simulink model "simu_test_2x1spokodziala1"  (Simulink 7.7)
settings: Solver=ode45  StartTime=0.0  StopTime=20.0  RelTol=1e-3
libraries: fuzblock x1, simulink x1
settings Model: Creator=Marcin  LastModifiedBy=Marcin

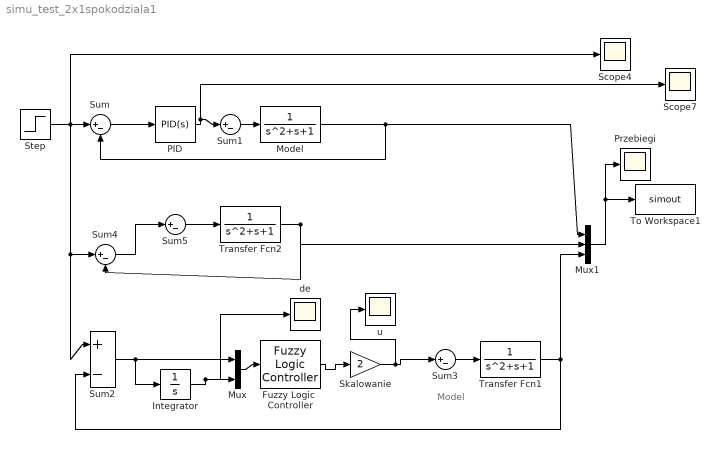
== system simu_test_2x1spokodziala1 ==
  note: Model
  Fuzzy Logic  Controller : fuzblock/Fuzzy Logic  Controller  SystemSampleTime=-1  fis=fls
  Integrator : Integrator
  Model : TransferFcn  Denominator=[1 1 1]
  Mux : Mux  Inputs=2
  Mux1 : Mux  Inputs=3
  PID : simulink/Continuous/PID Controller  SystemSampleTime=-1  Controller=PID  TimeDomain=Continuous-time  SampleTime=1  IntegratorMethod=Forward Euler  FilterMethod=Forward Euler  Form=Parallel  P=1  I=0.3  D=1  N=100  InitialConditionSource=internal  InitialConditionForIntegrator=0  InitialConditionForFilter=0  ExternalReset=none  LimitOutput=off  UpperSaturationLimit=inf  LowerSaturationLimit=-inf  LinearizeAsGain=off  AntiWindupMode=none  Kb=1  TrackingMode=off  Kt=1  PParamMin=[]  PParamMax=[]  IParamMin=[]  IParamMax=[]  DParamMin=[]  DParamMax=[]  NParamMin=[]  NParamMax=[]  KbParamMin=[]  KbParamMax=[]  KtParamMin=[]  KtParamMax=[]  POutMin=[]  POutMax=[]  IOutMin=[]  IOutMax=[]  DOutMin=[]  DOutMax=[]  NOutMin=[]  NOutMax=[]  KbOutMin=[]  KbOutMax=[]  KtOutMin=[]  KtOutMax=[]  IntegratorOutMin=[]  IntegratorOutMax=[]  FilterOutMin=[]  FilterOutMax=[]  SumOutMin=[]  SumOutMax=[]  SumI1OutMin=[]  SumI1OutMax=[]  SumI2OutMin=[]  SumI2OutMax=[]  SumI3OutMin=[]  SumI3OutMax=[]  SumDOutMin=[]  SumDOutMax=[]  SaturationOutMin=[]  SaturationOutMax=[]  IntegratorContinuousStateAttributes=''  IntegratorStateMustResolveToSignalObject=off  IntegratorRTWStateStorageClass=Auto  FilterContinuousStateAttributes=''  FilterStateMustResolveToSignalObject=off  FilterRTWStateStorageClass=Auto
  Przebiegi : Scope
      settings: TimeRange=20  YMin=0.45  YMax=1
  Scope4 : Scope
      settings: SaveName=ScopeData4
  Scope7 : Scope
      settings: YMin=0.3  YMax=0.95  SaveName=ScopeData7
  Skalowanie : Gain  Gain=2
  Step : Step  SampleTime=0
  Sum{,1..5} (6 alike) : Sum  Inputs=|+-
  To Workspace1 : ToWorkspace  VariableName=simout  SampleTime=-1  SaveFormat=Structure
  Transfer Fcn1 : TransferFcn  Denominator=[1 1 1]
  Transfer Fcn2 : TransferFcn  Numerator=1  Denominator=[1 1 1]
  de : Scope
      settings: YMin=1.01075  YMax=1.01425  SaveName=ScopeData5
  u : Scope
      settings: YMin=0  YMax=1.3  SaveName=ScopeData6
  wires:
  Sum/1 -> PID/1
  Model/1 -> Sum/2, Mux1/1
  Step/1 -> Sum/1, Sum4/1, Sum2/1, Scope4/1
  PID/1 -> Sum1/1, Scope7/1
  Sum1/1 -> Model/1
  Transfer Fcn1/1 -> Sum2/2, Mux1/3
  Mux/1 -> Fuzzy Logic  Controller/1
  Transfer Fcn2/1 -> Sum4/2, Mux1/2
  Mux1/1 -> Przebiegi/1, To Workspace1/1
  Fuzzy Logic  Controller/1 -> Skalowanie/1
  Sum2/1 -> Mux/1, Integrator/1
  Integrator/1 -> Mux/2, de/1
  Skalowanie/1 -> Sum3/1, u/1
  Sum3/1 -> Transfer Fcn1/1
  Sum5/1 -> Transfer Fcn2/1
  Sum4/1 -> Sum5/1
